simulink subsystem "L1_Adaptive_Controller"  (R2024a)
settings: Solver=VariableStepAuto  StartTime=0.0  StopTime=10.0  RelTol=1e-3
undefined symbols (not defined in the file): L1, Sim, vehicle
libraries: eeGeneralControl x3
settings Model: Creator=gurt1  LastModifiedBy=gurt1

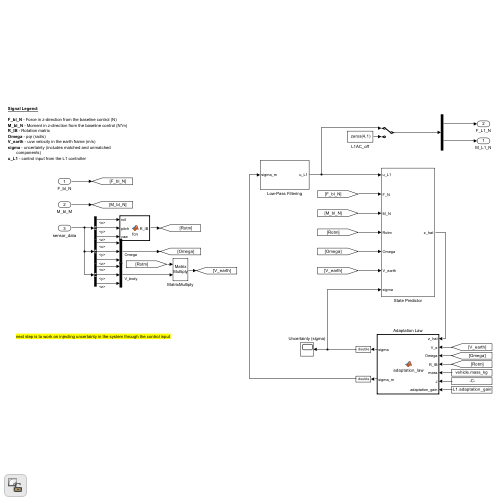
[thumbnail: Simulink's stored preview of the top-level diagram]
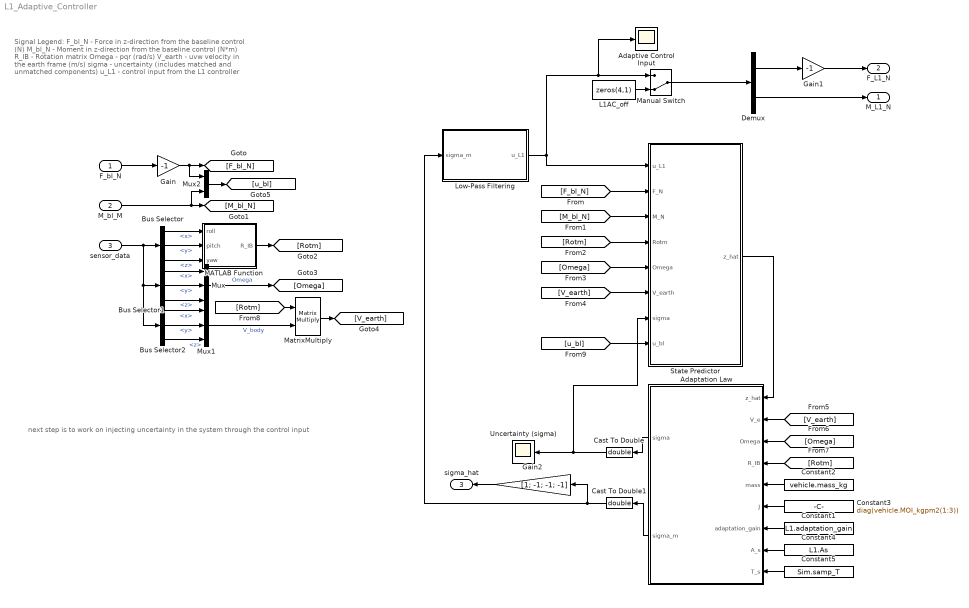
== system L1_Adaptive_Controller ==
  note: next step is to work on injecting uncertainty in the system through the control input
  note: Signal Legend:
      |
      | F_bl_N - Force in z-direction from the baseline control (N)
      | M_bl_N - Moment in z-direction from the baseline control (N*m)
      | R_IB - Rotation matrix
      | Omega - pqr (rad/s)
      | V_earth - uvw velocity in the earth frame (m/s)
      | sigma - uncertainty (includes matched and unmatched components)
      | u_L1 - control input from the L1 controller
  F_bl_N : Inport
  M_bl_M : Inport  Port=2
  sensor_data : Inport  Port=3
  Adaptation Law : MATLAB Function  TreatAsAtomicUnit=on
  Adaptive Control Input : Scope
  Bus Selector : BusSelector  OutputSignals=att_rad.x,att_rad.y,att_rad.z
  Bus Selector1 : BusSelector  OutputSignals=ang_rps.x,ang_rps.y,ang_rps.z
  Bus Selector2 : BusSelector  OutputSignals=vel_ned_mps.x,vel_ned_mps.y,vel_ned_mps.z
  Cast To Double : DataTypeConversion  OutDataTypeStr=double  SaturateOnIntegerOverflow=off  RndMeth=Floor
  Cast To Double1 : DataTypeConversion  OutDataTypeStr=double  SaturateOnIntegerOverflow=off  RndMeth=Floor
  Constant1 : Constant  Value=L1.adaptation_gain
  Constant2 : Constant  Value=vehicle.mass_kg
  Constant3 : Constant  Value=diag(vehicle.MOI_kgpm2(1:3))
  Constant4 : Constant  Value=L1.As
  Constant5 : Constant  Value=Sim.samp_T
  Demux : Demux  Outputs=[1 3]
  Gain : Gain  Gain=-1
  Gain1 : Gain  Gain=-1
  Gain2 : Gain  Gain=[1; -1; -1; -1]
  L1AC_off : Constant  Value=zeros(4,1)
  Low-Pass Filtering : Subsystem
  MATLAB Function : MATLAB Function  TreatAsAtomicUnit=on
  Manual Switch : ManualSwitch  CurrentSetting=0
  MatrixMultiply : Product  Multiplication=Matrix(*)
  Mux : Mux  Inputs=3
  Mux1 : Mux  Inputs=3
  Mux2 : Mux  Inputs=2
  State Predictor : Subsystem
  Uncertainty (sigma) : Scope
  M_L1_N : Outport
  F_L1_N : Outport  Port=2
  sigma_hat : Outport  Port=3
  wires:
  sensor_data/1 -> Bus Selector/1, Bus Selector1/1, Bus Selector2/1
  Bus Selector/1 -> MATLAB Function/1(roll)  "<x>"
  Bus Selector/2 -> MATLAB Function/2(pitch)  "<y>"
  Bus Selector/3 -> MATLAB Function/3(yaw)  "<z>"
  Bus Selector1/1 -> Mux/1  "<x>"
  Bus Selector1/2 -> Mux/2  "<y>"
  Bus Selector1/3 -> Mux/3  "<z>"
  Bus Selector2/1 -> Mux1/1  "<x>"
  Bus Selector2/2 -> Mux1/2  "<y>"
  Bus Selector2/3 -> Mux1/3  "<z>"
  F_bl_N/1 -> Gain/1
  M_bl_M/1 -> [M_bl_N], Mux2/2
  [F_bl_N] -> State Predictor/2(F_N)
  [M_bl_N] -> State Predictor/3(M_N)
  MATLAB Function/1(R_IB) -> [Rotm]
  Mux/1 -> [Omega]  "Omega"
  [Rotm] -> State Predictor/4(Rotm)
  [Omega] -> State Predictor/5(Omega)
  [V_earth] -> State Predictor/6(V_earth)
  State Predictor/1(z_hat) -> Adaptation Law/1(z_hat)
  [V_earth] -> Adaptation Law/2(V_e)
  [Omega] -> Adaptation Law/3(Omega)
  [Rotm] -> Adaptation Law/4(R_IB)
  Adaptation Law/1(sigma) -> Cast To Double/1
  Cast To Double/1 -> Uncertainty (sigma)/1, State Predictor/7(sigma)
  Adaptation Law/2(sigma_m) -> Cast To Double1/1
  Low-Pass Filtering/1(u_L1) -> State Predictor/1(u_L1), Manual Switch/1, Adaptive Control Input/1
  Demux/1 -> Gain1/1
  Demux/2 -> M_L1_N/1
  Cast To Double1/1 -> Gain2/1, Low-Pass Filtering/1(sigma_m)
  Constant3/1 -> Adaptation Law/6(J)
  Constant1/1 -> Adaptation Law/7(adaptation_gain)
  MatrixMultiply/1 -> [V_earth]
  [Rotm] -> MatrixMultiply/1
  Mux1/1 -> MatrixMultiply/2  "V_body"
  Manual Switch/1 -> Demux/1
  L1AC_off/1 -> Manual Switch/2
  Constant2/1 -> Adaptation Law/5(mass)
  Gain/1 -> [F_bl_N], Mux2/1
  Gain1/1 -> F_L1_N/1
  Gain2/1 -> sigma_hat/1
  Mux2/1 -> [u_bl]
  [u_bl] -> State Predictor/8(u_bl)
  Constant4/1 -> Adaptation Law/8(A_s)
  Constant5/1 -> Adaptation Law/9(T_s)

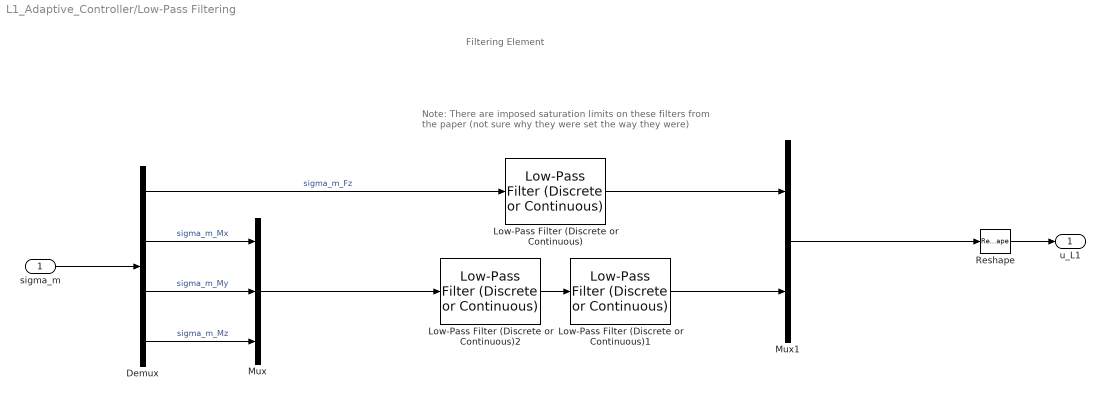
== system L1_Adaptive_Controller/Low-Pass Filtering ==
  note: Note:
      | There are imposed saturation limits on these filters from the paper (not sure why they were set the way they were)
  note: Filtering Element
  sigma_m : Inport
  Demux : Demux
  Low-Pass Filter (Discrete or Continuous) : eeGeneralControl/Low-Pass Filter (Discrete or Continuous)  K=1  T=1/12  B=inf  A=-inf  init_option=Specify as parameter  x0=0  Ts=-1
  Low-Pass Filter (Discrete or Continuous)1 : eeGeneralControl/Low-Pass Filter (Discrete or Continuous)  K=1  T=1/4  B=inf  A=-inf  init_option=Specify as parameter  x0=0  Ts=-1
  Low-Pass Filter (Discrete or Continuous)2 : eeGeneralControl/Low-Pass Filter (Discrete or Continuous)  K=1  T=1/6  B=inf  A=-inf  init_option=Specify as parameter  x0=0  Ts=-1
  Mux : Mux  Inputs=3
  Mux1 : Mux  Inputs=2
  Reshape : Reshape
  u_L1 : Outport
  wires:
  Mux1/1 -> Reshape/1
  Reshape/1 -> u_L1/1
  Low-Pass Filter (Discrete or Continuous)/1 -> Mux1/1
  Low-Pass Filter (Discrete or Continuous)1/1 -> Mux1/2
  Low-Pass Filter (Discrete or Continuous)2/1 -> Low-Pass Filter (Discrete or Continuous)1/1
  Mux/1 -> Low-Pass Filter (Discrete or Continuous)2/1
  Demux/1 -> Low-Pass Filter (Discrete or Continuous)/1  "sigma_m_Fz"
  Demux/2 -> Mux/1  "sigma_m_Mx"
  Demux/3 -> Mux/2  "sigma_m_My"
  Demux/4 -> Mux/3  "sigma_m_Mz"
  sigma_m/1 -> Demux/1

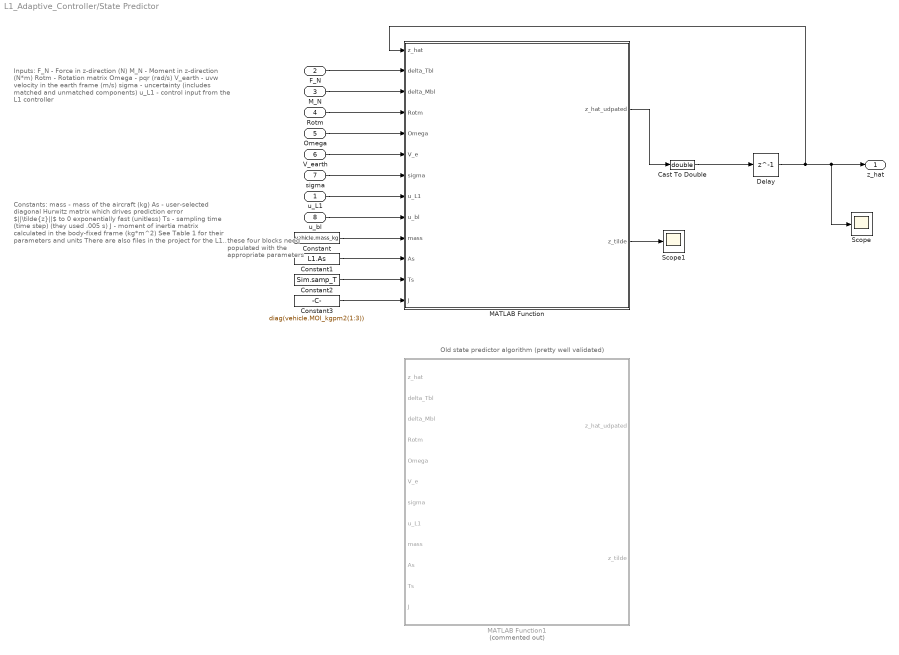
== system L1_Adaptive_Controller/State Predictor ==
  note: Inputs:
      |
      | F_N - Force in z-direction (N)
      | M_N - Moment in z-direction (N*m)
      | Rotm - Rotation matrix
      | Omega - pqr (rad/s)
      | V_earth - uvw velocity in the earth frame (m/s)
      | sigma - uncertainty (includes matched and unmatched components)
      | u_L1 - control input from the L1 controller
  note: Constants:
      | mass - mass of the aircraft (kg)
      | As - user-selected diagonal Hurwitz
      | matrix which drives prediction error $||\tilde{z}||$ to 0 exponentially fast (unitless)
      | Ts - sampling time (time step) (they used .005 s)
      | J - moment of inertia matrix calculated in the body-fixed frame (kg*m^2)
      |
      | See Table 1 for their parameters and units
      |
      | There are also files in the project for the L1 quad paper that have these variables defined if there is confusion
  note: these four blocks need populated with the appropriate parameters
  note: Old state predictor algorithm (pretty well validated)
  u_L1 : Inport
  F_N : Inport  Port=2
  M_N : Inport  Port=3
  Rotm : Inport  Port=4
  Omega : Inport  Port=5
  V_earth : Inport  Port=6
  sigma : Inport  Port=7
  u_bl : Inport  Port=8
  Cast To Double : DataTypeConversion  OutDataTypeStr=double  SaturateOnIntegerOverflow=off  RndMeth=Floor
  Constant : Constant  Value=vehicle.mass_kg
  Constant1 : Constant  Value=L1.As
  Constant2 : Constant  Value=Sim.samp_T
  Constant3 : Constant  Value=diag(vehicle.MOI_kgpm2(1:3))
  Delay : Delay  DelayLength=1  InitialCondition=[0 0 0 0 0 0]
  MATLAB Function : MATLAB Function  TreatAsAtomicUnit=on
  MATLAB Function1 : MATLAB Function  Commented=on  TreatAsAtomicUnit=on
  Scope : Scope
  Scope1 : Scope
  z_hat : Outport
  wires:
  u_bl/1 -> MATLAB Function/9(u_bl)
  MATLAB Function/2(z_tilde) -> Scope1/1
  Constant1/1 -> MATLAB Function/11(As)
  Constant2/1 -> MATLAB Function/12(Ts)
  Constant3/1 -> MATLAB Function/13(J)
  Constant/1 -> MATLAB Function/10(mass)
  sigma/1 -> MATLAB Function/7(sigma)
  F_N/1 -> MATLAB Function/2(delta_Tbl)
  M_N/1 -> MATLAB Function/3(delta_Mbl)
  V_earth/1 -> MATLAB Function/6(V_e)
  Omega/1 -> MATLAB Function/5(Omega)
  Rotm/1 -> MATLAB Function/4(Rotm)
  u_L1/1 -> MATLAB Function/8(u_L1)
  Delay/1 -> MATLAB Function/1(z_hat), z_hat/1, Scope/1
  Cast To Double/1 -> Delay/1
  MATLAB Function/1(z_hat_udpated) -> Cast To Double/1

== matlab function L1_Adaptive_Controller/State Predictor/MATLAB Function1 ==
  data: z_hat input; delta_Tbl input; delta_Mbl input; Rotm input; Omega input; z_hat_udpated output; V_e input; sigma input; u_L1 input; mass input; As input; Ts input; J input; z_tilde output
function [z_hat_udpated, z_tilde]  = state_predictor(z_hat,delta_Tbl,delta_Mbl,Rotm,Omega,V_e,sigma,u_L1, mass, As, Ts, J)

% INPUTS
%
% z_hat -       Current state prediction (R6)
% delta_Tbl -   Force commanded from baseline control (1x1) [kg]
% delta_Mbl -   Moment commanded from baseline control (3x1) [kg*m^2]
% Rotm -        Rotation matrix calculated by Euler angles
% Omega -       Angular rates (p,q,r) [rad/s]
% V_e -         Velocity in the earth-fixed frame [m/s]
% sigma -       Uncertainty [matched (R4) unmatched (R2)]
% u_L1 -        Control input due to the L1 adaptive control
% mass -        Vehicle mass [kg]
% As -          User-selectable diagonal Hurwitz matrix that drives  
%               prediction error to $||\tilde{z}||$ to 0
% Ts -          Sample Time (interval) [s]
% J -           Diagonal moment of inertia matrix [kg*m^2]
% 
% OUTPUTS
%
% z_hat_updated - updated state prediction

b1 = Rotm(:,1);
b2 = Rotm(:,2);
b3 = Rotm(:,3);
e3 = [0;0;1];
sigma_m = sigma(1:4); % matched uncertainty
sigma_um = sigma(5:6); % unmatched uncertainty 
m = mass;

% f from the paper 
 fk = [ 9.81 * e3 + 1/m * delta_Tbl * b3;
       inv(J) * delta_Mbl - inv(J)*cross(Omega,J*Omega)];

% ????? Why is fk above the way that it is (see just f(z) in the paper) and
% what exactly is delta_Thrust_baseline and delta_Moment_baseline?

% B from the paper
 gk = [1/m * b3 , zeros(3,3);
      zeros(3,1) , inv(J)    ];   

% B^{perpendicular} from paper
gkp = [1/m * b1 , 1/m * b2;
        zeros(3,2)];

% State Predictor

% z_tilde - prediction error (predicted - actual)
z = [V_e;Omega]; % Actual state of the system
z_tilde = z_hat - z; % Error in state prediction ($\tilde{z}$)

% Equation (7) for $\dot{\hat{z}}$ for the state predictor was integrated,
% multiplied by the sample time, and is added to the old value of z_hat to
% yield an updated value for z_hat (the state estimate)
z_hat_udpated = z_hat + [fk + gk * (u_L1 + sigma_m) + gkp * sigma_um + As * z_tilde] * Ts;

% zkupdate = zk + [fk + As * zk_wiggle] * Ts;function y = fcn(u)

== matlab function L1_Adaptive_Controller/MATLAB Function ==
  data: roll input; pitch input; yaw input; R_IB output
function R_IB = fcn(roll, pitch, yaw)

R_IB = eul2rotm([yaw pitch roll]);

== matlab function L1_Adaptive_Controller/State Predictor/MATLAB Function ==
  data: z_hat input; delta_Tbl input; delta_Mbl input; Rotm input; Omega input; z_hat_udpated output; V_e input; sigma input; u_L1 input; u_bl input; mass input; As input; Ts input; J input; z_tilde output
function [z_hat_udpated, z_tilde]  = state_predictor(z_hat,delta_Tbl,delta_Mbl,Rotm,Omega,V_e,sigma,u_L1,u_bl, mass, As, Ts, J)

% INPUTS
%
% z_hat -       Current state prediction (R6)
% delta_Tbl -   Force commanded from baseline control (1x1) [kg]
% delta_Mbl -   Moment commanded from baseline control (3x1) [kg*m^2]
% Rotm -        Rotation matrix calculated by Euler angles
% Omega -       Angular rates (p,q,r) [rad/s]
% V_e -         Velocity in the earth-fixed frame [m/s]
% sigma -       Uncertainty [matched (R4) unmatched (R2)]
% u_L1 -        Control input due to the L1 adaptive control
% mass -        Vehicle mass [kg]
% As -          User-selectable diagonal Hurwitz matrix that drives  
%               prediction error to $||\tilde{z}||$ to 0
% Ts -          Sample Time (interval) [s]
% J -           Diagonal moment of inertia matrix [kg*m^2]
% 
% OUTPUTS
%
% z_hat_updated - updated state prediction

b1 = Rotm(:,1);
b2 = Rotm(:,2);
b3 = Rotm(:,3);
e3 = [0;0;1];
sigma_m = sigma(1:4); % matched uncertainty
sigma_um = sigma(5:6); % unmatched uncertainty 
m = mass;

% Old formulation of f from the paper 
% (**NOTE** It already accounts for u_bl but works it into the f matrix, 
% so if using this, use the version of z_hat_updated that doesn't include u_bl)
 % fk = [ 9.81 * e3 + 1/m * delta_Tbl * b3;
 %       inv(J) * delta_Mbl - inv(J)*cross(Omega,J*Omega)];

% ????? Why is fk above the way that it is (see just f(z) in the paper) and
% what exactly is delta_Thrust_baseline and delta_Moment_baseline?

% B from the paper
 B = [1/m * b3 , zeros(3,3);
      zeros(3,1) , inv(J)];   

% B^{perpendicular} from paper
B_perp = [1/m * b1 , 1/m * b2;
        zeros(3,2)];

% State Predictor

% z_tilde - prediction error (predicted - actual)
z = [V_e;Omega]; % Actual state of the system
z_tilde = z_hat - z; % Error in state prediction ($\tilde{z}$)

% Equation (7) for $\dot{\hat{z}}$ for the state predictor was integrated,
% multiplied by the sample time, and is added to the old value of z_hat to
% yield an updated value for z_hat (the state estimate)
% Old one (validated)
%z_hat_udpated = z_hat + [fk + B * (u_L1 + sigma_m) + B_perp * sigma_um + As * z_tilde] * Ts;


% NEW EXPERIMENTAL FORMULATIONS
fk = [9.81*e3; inv(J)*cross(Omega,J*Omega)];

% New one (validation in progress)
z_hat_udpated = z_hat + [fk + B * (u_bl + u_L1 + sigma_m) + B_perp * sigma_um + As * z_tilde] * Ts;

== matlab function L1_Adaptive_Controller/Adaptation Law ==
  data: z_hat input; V_e input; sigma output; Omega input; R_IB input; mass input; sigma_m output; J input; adaptation_gain input; A_s input; T_s input
function [sigma, sigma_m] = adaptation_law(z_hat, V_e, Omega, R_IB, mass, J, adaptation_gain, A_s, T_s)

% INPUTS
%
% z_hat -       Current state prediction (6x1)
% V_e -         Velocity in the earth-fixed frame [m/s]
% Omega -       Angular rates (p,q,r) [rad/s]
% Rotm -        Rotation matrix calculated by Euler angles (3x3)
% J -           Diagonal moment of inertia matrix [kg*m^2]
% adaptation_gain - Set externally in the controller initialization
% 
% OUTPUTS
% sigma - uncertainty [Fz,Mx,My,Mz,Fx,Fy] (matched & unmatched)
% sigma_m - matched uncertainty in [Fz,Mx,My,Mz] respectively 

b1 = R_IB(:,1);
b2 = R_IB(:,2);
b3 = R_IB(:,3);
m = mass;

% Precomputed B_bar_inv from the paper
B_bar_inv = [m*b3', zeros(1,3);
            zeros(3,3), J;
            m*b1', zeros(1,3);
            m*b2', zeros(1,3)];
ind = eye(6);
z = [V_e; Omega]; % actual reduced system state
z_tilde = z_hat - z; % state prediction error

% % New formulation
%  B = [1/m * b3 , zeros(3,3);
%       zeros(3,1) , inv(J)    ];  
% 
% % B^{perpendicular} from paper
% B_perp = [1/m * b1 , 1/m * b2;
%         zeros(3,2)];
% 
% B_bar = [B, B_perp];
% B_bar_inv = inv(B_bar);

% New formulation for output
%sigma = -eye(6)*B_bar_inv*(exp(A_s*T_s)-eye(6))^(-1)*A_s*exp(A_s*T_s)*(z_tilde);
%sigma = -B_bar_inv*(exp(A_s*T_s)-eye(6))^(-1)*A_s*exp(A_s*T_s)*(z_tilde);
%sigma_m = -sigma(1:4);

% Old uncertainty calculations (sigma) that worked
% Note: these match the formulations presented in their 2023 archive paper
sigma = -ind*B_bar_inv*adaptation_gain*(z_tilde);
sigma_m = -sigma(1:4);
